simulink model "vending"  (R2020b)
settings: Solver=VariableStepAuto  StartTime=0.0  StopTime=200  RelTol=1e-3
settings Model: EnablePacing=on  PacingRate=4  Creator=shivanshu shukla  LastModifiedBy=shivanshu shukla

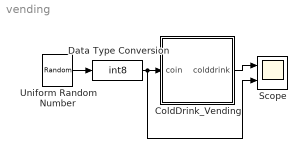
== system vending ==
  ColdDrink_Vending : Stateflow chart  TreatAsAtomicUnit=on
  Data Type Conversion : DataTypeConversion  OutDataTypeStr=int8  RndMeth=Nearest
  Scope : Scope  NumInputPorts=2
  Uniform Random Number : UniformRandomNumber  Minimum=0  Maximum=2  Seed=337  SampleTime=10
  wires:
  Uniform Random Number/1 -> Data Type Conversion/1
  Data Type Conversion/1 -> Scope/2, ColdDrink_Vending/1(coin)
  ColdDrink_Vending/1(colddrink) -> Scope/1

== stateflow chart vending/ColdDrink_Vending ==
  settings: stateMachineType=MEALY_MACHINE  initializeOutput=1
  state got_0
  state got_50note
  state got_100note
  (default) -> got_0
  got_0 -> got_50note [order 1] : [coin==1]{colddrink=0}
  got_50note -> got_0 [order 2] : [coin==2]{colddrink=1}
  got_100note -> got_0 [order 1] : [coin==1]{colddrink=1}
  got_0 -> got_100note [order 2] : [coin==2]{colddrink=0}
  got_50note -> got_100note [order 1] : [coin==1]{colddrink=0}
  got_100note -> got_50note [order 2] : [coin==2]{colddrink=1}
  data: colddrink output boolean [0..1]; coin input int8
